simulink model "chap7_7sim"  (Simulink 8.1)
settings: Solver=ode45  StartTime=0.0  StopTime=10  FixedStep=0.001  RelTol=1e-3
settings Model: Creator=hp  LastModifiedBy=liujk
settings OptimizationCC: InitFltsAndDblsToZero=on
settings DebuggingCC: SaveWithParameterizedLinksMsg=none  SignalResolutionControl=TryResolveAllWithWarning  SolverPrmCheckMsg=none  MultiTaskDSMMsg=warning  MultiTaskCondExecSysMsg=none  StrictBusMsg=Warning
settings RTWCC: IncludeERTFirstTime=on
settings GRTTargetCC: TargetFcnLib=ansi_tfl_tmw.mat

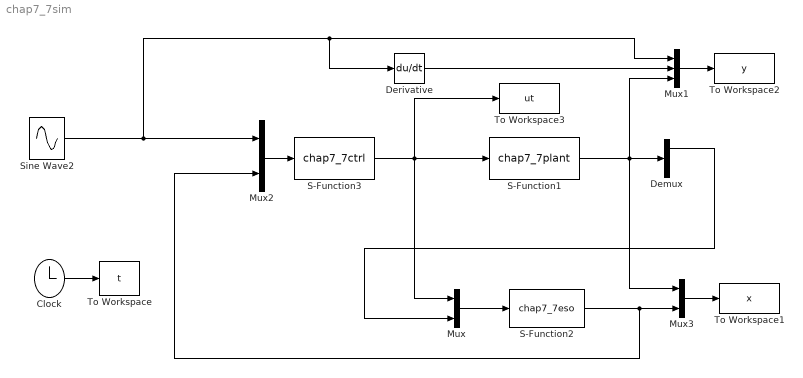
== system chap7_7sim ==
  Clock : Clock
      settings: Decimation=30
  Demux : Demux  Outputs=3
  Derivative : Derivative
  Mux : Mux  Inputs=2
  Mux1 : Mux  Inputs=3
  Mux2 : Mux  Inputs=2
  Mux3 : Mux  Inputs=2
  S-Function1 : S-Function  FunctionName=chap7_7plant  EnableBusSupport=off
  S-Function2 : S-Function  FunctionName=chap7_7eso  EnableBusSupport=off
  S-Function3 : S-Function  FunctionName=chap7_7ctrl  EnableBusSupport=off
  Sine Wave2 : Sin  SampleTime=0
  To Workspace : ToWorkspace  VariableName=t  SampleTime=-1
  To Workspace1 : ToWorkspace  VariableName=x  SampleTime=-1
  To Workspace2 : ToWorkspace  VariableName=y  SampleTime=-1
  To Workspace3 : ToWorkspace  VariableName=ut  SampleTime=-1
  wires:
  Clock/1 -> To Workspace/1
  Sine Wave2/1 -> Mux1/1, Derivative/1, Mux2/1
  S-Function3/1 -> S-Function1/1, To Workspace3/1, Mux/1
  Mux/1 -> S-Function2/1
  Mux1/1 -> To Workspace2/1
  Mux2/1 -> S-Function3/1
  S-Function2/1 -> Mux3/2, Mux2/2
  S-Function1/1 -> Demux/1, Mux1/3, Mux3/1
  Demux/1 -> Mux/2
  Mux3/1 -> To Workspace1/1
  Derivative/1 -> Mux1/2
